simulink model "MainSim"  (R2024a)
(part 10 of 12)

  "IW{1,1}(91,:)'" : Constant  Value=[0.07063741223789991863224457802061806432902812957763671875;-0.08871882270486421140365251858383999206125736236572265625;0.0006579027296117509297779246679738207603804767131805419921875;-0.01173923498918761666731658266371596255339682102203369140625;-0.01047479372654045760848706692058840417303144931793212890625;-0.019136290652363503739241679113547434099018573760986328125;-0.0260832109095130472431467438809704617597162723541259765625;0.0247262166900140654968165421223602606914937496185302734375;-0.0230945968221924653740462218820539419539272785186767578125;-0.00669175803018199656657660767677953117527067661285400390625;-0.02521354944576546797119220855165622197091579437255859375;0.00151431210226198845365808143270669461344368755817413330078125;0.02841805038105411906901309748718631453812122344970703125;0.0267906724159141622354507461523098754696547985076904296875]
      mask Display: e = 0.06;c1 = [120 150 230]/255;c2 = ([120 150 230]+0)/383;c3 = ([120 150 230]+128)/383;patch([0 1 1 0],[0 0 1 1],c1);patch([0 1 1 1-e 1-e 0+e],[0 0 1 1-e 0+e 0+e],c2);patch([0 0 1 1-e 0+e 0+e],[0 1 1 1-e 1-e 0+e],c3);plot([0 1 1 0 0],[0 0 1 1 0]);disp('Weights');
  "IW{1,1}(92,:)'" : Constant  Value=[-0.01208219342854178167401268950698067783378064632415771484375;0.0067192472598249473880738236175602651201188564300537109375;-0.01018004902194633194689732391680081491358578205108642578125;-0.0034201050886383775606613966147051542066037654876708984375;-0.00346664875944259487372534067617380060255527496337890625;0.00407538024919248086097578465114565915428102016448974609375;-0.0001579382642456296005108173918785041678347624838352203369140625;0.004590930287056878278395544157319818623363971710205078125;-0.006531130622358559227602636809706382337026298046112060546875;-0.007838052866014667829919204677935340441763401031494140625;0.01154164356092016695265467518538571312092244625091552734375;-0.00469984162117397137603536094729861360974609851837158203125;0.0053619108677808897944760957443577353842556476593017578125;0.0128726196335035812656766296413479722104966640472412109375]
      mask Display: e = 0.06;c1 = [120 150 230]/255;c2 = ([120 150 230]+0)/383;c3 = ([120 150 230]+128)/383;patch([0 1 1 0],[0 0 1 1],c1);patch([0 1 1 1-e 1-e 0+e],[0 0 1 1-e 0+e 0+e],c2);patch([0 0 1 1-e 0+e 0+e],[0 1 1 1-e 1-e 0+e],c3);plot([0 1 1 0 0],[0 0 1 1 0]);disp('Weights');
  "IW{1,1}(93,:)'" : Constant  Value=[0.00663469289612939223943488542545310338027775287628173828125;-0.0029780897264123393046453269761286719585768878459930419921875;0.005417420119265266113817158810661567258648574352264404296875;0.00455848440464646890990518812714071827940642833709716796875;0.0019560567513700354881633902692783522070385515689849853515625;-0.00565136530838120619557596313597969128750264644622802734375;-0.010249816397415255353475771471494226716458797454833984375;0.00870667414768099001687318150288774631917476654052734375;-0.00642539976546986808803030299941383418627083301544189453125;0.00147365805093719660391615722261349219479598104953765869140625;0.0065425459944154218394629651811555959284305572509765625;0.00208761620669374418912678237347790854983031749725341796875;-0.00134558529696151532757675273188624487374909222126007080078125;0.006577099244312635539788658434190438129007816314697265625]
      mask Display: e = 0.06;c1 = [120 150 230]/255;c2 = ([120 150 230]+0)/383;c3 = ([120 150 230]+128)/383;patch([0 1 1 0],[0 0 1 1],c1);patch([0 1 1 1-e 1-e 0+e],[0 0 1 1-e 0+e 0+e],c2);patch([0 0 1 1-e 0+e 0+e],[0 1 1 1-e 1-e 0+e],c3);plot([0 1 1 0 0],[0 0 1 1 0]);disp('Weights');
  "IW{1,1}(94,:)'" : Constant  Value=[0.0133196975876473978905867312505506561137735843658447265625;-0.002724954991086264190214283331670230836607515811920166015625;-0.01292568993384780352828844485202353098429739475250244140625;-0.00010258642474367216947638004054255134178674779832363128662109375;0.0034192712014378713603068860038547427393496036529541015625;-0.0049133132011409709483107377536725834943354129791259765625;-0.0214623812474793208837642310982118942774832248687744140625;0.023007485850688368100858127718311152420938014984130859375;0.019016587387684143195532016079596360214054584503173828125;0.0058914858069833986320418262039311230182647705078125;0.0019757847315106220019431670920084798126481473445892333984375;0.0001740592937999706885619788376828864784329198300838470458984375;-0.005836771553343969749783060052550354157574474811553955078125;-0.01172118802567679619885954167557429173029959201812744140625]
      mask Display: e = 0.06;c1 = [120 150 230]/255;c2 = ([120 150 230]+0)/383;c3 = ([120 150 230]+128)/383;patch([0 1 1 0],[0 0 1 1],c1);patch([0 1 1 1-e 1-e 0+e],[0 0 1 1-e 0+e 0+e],c2);patch([0 0 1 1-e 0+e 0+e],[0 1 1 1-e 1-e 0+e],c3);plot([0 1 1 0 0],[0 0 1 1 0]);disp('Weights');
  "IW{1,1}(95,:)'" : Constant  Value=[-0.030168984435360361728850620011144201271235942840576171875;-0.00242856335944273242499757969881102326326072216033935546875;0.045366474304561275887603954970472841523587703704833984375;0.0235956203780624991506176257871629786677658557891845703125;0.0088950917664759772407467863786223460920155048370361328125;-0.04038602680676041389862263031318434514105319976806640625;-0.055396583699348807272588857131268014200031757354736328125;0.034673033558393163977573436795864836312830448150634765625;-0.01259596599131877769917053910830873064696788787841796875;0.00887435102632798920863077540843733004294335842132568359375;0.021710772551334543700729540205429657362401485443115234375;-0.01202374062881248449607962669460903271101415157318115234375;-0.00913509215609213144626554736760226660408079624176025390625;0.020010212544438167603377820569221512414515018463134765625]
      mask Display: e = 0.06;c1 = [120 150 230]/255;c2 = ([120 150 230]+0)/383;c3 = ([120 150 230]+128)/383;patch([0 1 1 0],[0 0 1 1],c1);patch([0 1 1 1-e 1-e 0+e],[0 0 1 1-e 0+e 0+e],c2);patch([0 0 1 1-e 0+e 0+e],[0 1 1 1-e 1-e 0+e],c3);plot([0 1 1 0 0],[0 0 1 1 0]);disp('Weights');
  "IW{1,1}(96,:)'" : Constant  Value=[-0.05226400603406648748272544935389305464923381805419921875;0.0273221261562778573728227371475441032089293003082275390625;0.0258205096419121642170591002241053502075374126434326171875;0.0113152954568486972808383228539241827093064785003662109375;-0.0110224380149167890119432655637865536846220493316650390625;-0.0183353680525855343430574606600202969275414943695068359375;-0.018711723571017128964211195807365584187209606170654296875;-0.0173876375265110405532453796695335768163204193115234375;0.00068990722089190830053351266570871302974410355091094970703125;0.02452344814787373039610685054867644794285297393798828125;-0.015917217658364547772098518407801748253405094146728515625;0.0109260537933429692503128904945697286166250705718994140625;0.006101429406713741905587955471901295823045074939727783203125;0.007714180790291681223680431145339753129519522190093994140625]
      mask Display: e = 0.06;c1 = [120 150 230]/255;c2 = ([120 150 230]+0)/383;c3 = ([120 150 230]+128)/383;patch([0 1 1 0],[0 0 1 1],c1);patch([0 1 1 1-e 1-e 0+e],[0 0 1 1-e 0+e 0+e],c2);patch([0 0 1 1-e 0+e 0+e],[0 1 1 1-e 1-e 0+e],c3);plot([0 1 1 0 0],[0 0 1 1 0]);disp('Weights');
  "IW{1,1}(97,:)'" : Constant  Value=[-0.01271120469215512686911306872161731007508933544158935546875;0.0029051811219069716661633773213679887703619897365570068359375;0.0026221018723518560618324091393560593132860958576202392578125;-0.005134367328952889157622774263245446491055190563201904296875;-0.00274391636624273828337639002938885823823511600494384765625;-0.008903427967942099952036727472659549675881862640380859375;-0.01394853375048086228937815889139528735540807247161865234375;0.0161885508909591878390354935390860191546380519866943359375;0.006177978217436277084961826489006853080354630947113037109375;-0.00474236355881050251903641168382819159887731075286865234375;0.0011100417623952272237752847416913937195204198360443115234375;-0.007804969943815354138649809101480059325695037841796875;0.0026443898432858318169047517898206933750770986080169677734375;-0.002549758171897571756847611368357320316135883331298828125]
      mask Display: e = 0.06;c1 = [120 150 230]/255;c2 = ([120 150 230]+0)/383;c3 = ([120 150 230]+128)/383;patch([0 1 1 0],[0 0 1 1],c1);patch([0 1 1 1-e 1-e 0+e],[0 0 1 1-e 0+e 0+e],c2);patch([0 0 1 1-e 0+e 0+e],[0 1 1 1-e 1-e 0+e],c3);plot([0 1 1 0 0],[0 0 1 1 0]);disp('Weights');
  "IW{1,1}(98,:)'" : Constant  Value=[0.01680988917533955684380231332397670485079288482666015625;-0.016287284319194537951513979123774333856999874114990234375;0.006126833448734378580191606289417904918082058429718017578125;0.00891914449581840580727476464062419836409389972686767578125;0.0052329151305931242976754447226994670927524566650390625;-0.0141034774720301403494460146248457022011280059814453125;-0.0241382135885616598558467416069106548093259334564208984375;0.01558620993734481825765403328887259704060852527618408203125;-0.00181381654274688866070042170264287051395513117313385009765625;0.00478300775746385957443163050584189477376639842987060546875;0.00464685931016431581774828174502545152790844440460205078125;0.00166038039346685039297779606926042106351815164089202880859375;0.00118738160556240983541098632514376731705851852893829345703125;0.005989139214336841772479136380979980458505451679229736328125]
      mask Display: e = 0.06;c1 = [120 150 230]/255;c2 = ([120 150 230]+0)/383;c3 = ([120 150 230]+128)/383;patch([0 1 1 0],[0 0 1 1],c1);patch([0 1 1 1-e 1-e 0+e],[0 0 1 1-e 0+e 0+e],c2);patch([0 0 1 1-e 0+e 0+e],[0 1 1 1-e 1-e 0+e],c3);plot([0 1 1 0 0],[0 0 1 1 0]);disp('Weights');
  "IW{1,1}(99,:)'" : Constant  Value=[0.00915866334388989143666659487053038901649415493011474609375;-0.0199881171056931726537353455341872177086770534515380859375;0.0292708625049807914797472818690948770381510257720947265625;0.0273509617718294718857752201301991590298712253570556640625;0.0171598449904944612420809590958015178330242633819580078125;0.00935099324310617076305707229266772628761827945709228515625;0.0188901316024791994518938764713311684317886829376220703125;-0.011542775357101166255890944967177347280085086822509765625;0.014954836457782456904386236828941036947071552276611328125;0.017637024589468898450039802128230803646147251129150390625;-0.0021220429574456164782680911429224579478614032268524169921875;0.0004286890763189841742179797545730934871244244277477264404296875;0.00048205508339510213557110862581112087354995310306549072265625;-0.017889644911831655005318708617778611369431018829345703125]
      mask Display: e = 0.06;c1 = [120 150 230]/255;c2 = ([120 150 230]+0)/383;c3 = ([120 150 230]+128)/383;patch([0 1 1 0],[0 0 1 1],c1);patch([0 1 1 1-e 1-e 0+e],[0 0 1 1-e 0+e 0+e],c2);patch([0 0 1 1-e 0+e 0+e],[0 1 1 1-e 1-e 0+e],c3);plot([0 1 1 0 0],[0 0 1 1 0]);disp('Weights');
  Mux : Mux  Inputs=125
      mask Display: e = 0.06;c1 = [120 150 230]/255;c2 = ([120 150 230]+0)/383;c3 = ([120 150 230]+128)/383;patch([0 1 1 0],[0 0 1 1],c1);patch([0 1 1 1-e 1-e 0+e],[0 0 1 1-e 0+e 0+e],c2);patch([0 0 1 1-e 0+e 0+e],[0 1 1 1-e 1-e 0+e],c3);plot([0 1 1 0 0],[0 0 1 1 0]);disp('Mux');
  dotprod{1..125} (125 alike) : neural/Weight Functions/dotprod
  "iz{1,1}" : Outport
      mask Display: e = 0.06;c1 = [120 230 180]/255;c2 = ([120 230 180]+0)/(256+128);c3 = ([120 230 180]+128)/(256+128);patch([0 1 1 0],[0 0 1 1],c1);patch([0 1 1 1-e 1-e 0+e],[0 0 1 1-e 0+e 0+e],c2);patch([0 0 1 1-e 0+e 0+e],[0 1 1 1-e 1-e 0+e],c3);plot([0 1 1 0 0],[0 0 1 1 0]);
  wires:
  Mux/1 -> "iz{1,1}"/1
  dotprod125/1 -> Mux/125
  "IW{1,1}(125,:)'"/1 -> dotprod125/1
  dotprod124/1 -> Mux/124
  "IW{1,1}(124,:)'"/1 -> dotprod124/1
  dotprod123/1 -> Mux/123
  "IW{1,1}(123,:)'"/1 -> dotprod123/1
  dotprod122/1 -> Mux/122
  "IW{1,1}(122,:)'"/1 -> dotprod122/1
  dotprod121/1 -> Mux/121
  "IW{1,1}(121,:)'"/1 -> dotprod121/1
  dotprod120/1 -> Mux/120
  "IW{1,1}(120,:)'"/1 -> dotprod120/1
  dotprod119/1 -> Mux/119
  "IW{1,1}(119,:)'"/1 -> dotprod119/1
  dotprod118/1 -> Mux/118
  "IW{1,1}(118,:)'"/1 -> dotprod118/1
  dotprod117/1 -> Mux/117
  "IW{1,1}(117,:)'"/1 -> dotprod117/1
  dotprod116/1 -> Mux/116
  "IW{1,1}(116,:)'"/1 -> dotprod116/1
  dotprod115/1 -> Mux/115
  "IW{1,1}(115,:)'"/1 -> dotprod115/1
  dotprod114/1 -> Mux/114
  "IW{1,1}(114,:)'"/1 -> dotprod114/1
  dotprod113/1 -> Mux/113
  "IW{1,1}(113,:)'"/1 -> dotprod113/1
  dotprod112/1 -> Mux/112
  "IW{1,1}(112,:)'"/1 -> dotprod112/1
  dotprod111/1 -> Mux/111
  "IW{1,1}(111,:)'"/1 -> dotprod111/1
  dotprod110/1 -> Mux/110
  "IW{1,1}(110,:)'"/1 -> dotprod110/1
  dotprod109/1 -> Mux/109
  "IW{1,1}(109,:)'"/1 -> dotprod109/1
  dotprod108/1 -> Mux/108
  "IW{1,1}(108,:)'"/1 -> dotprod108/1
  dotprod107/1 -> Mux/107
  "IW{1,1}(107,:)'"/1 -> dotprod107/1
  dotprod106/1 -> Mux/106
  "IW{1,1}(106,:)'"/1 -> dotprod106/1
  dotprod105/1 -> Mux/105
  "IW{1,1}(105,:)'"/1 -> dotprod105/1
  dotprod104/1 -> Mux/104
  "IW{1,1}(104,:)'"/1 -> dotprod104/1
  dotprod103/1 -> Mux/103
  "IW{1,1}(103,:)'"/1 -> dotprod103/1
  dotprod102/1 -> Mux/102
  "IW{1,1}(102,:)'"/1 -> dotprod102/1
  dotprod101/1 -> Mux/101
  "IW{1,1}(101,:)'"/1 -> dotprod101/1
  dotprod100/1 -> Mux/100
  "IW{1,1}(100,:)'"/1 -> dotprod100/1
  dotprod99/1 -> Mux/99
  "IW{1,1}(99,:)'"/1 -> dotprod99/1
  dotprod98/1 -> Mux/98
  "IW{1,1}(98,:)'"/1 -> dotprod98/1
  dotprod97/1 -> Mux/97
  "IW{1,1}(97,:)'"/1 -> dotprod97/1
  dotprod96/1 -> Mux/96
  "IW{1,1}(96,:)'"/1 -> dotprod96/1
  dotprod95/1 -> Mux/95
  "IW{1,1}(95,:)'"/1 -> dotprod95/1
  dotprod94/1 -> Mux/94
  "IW{1,1}(94,:)'"/1 -> dotprod94/1
  dotprod93/1 -> Mux/93
  "IW{1,1}(93,:)'"/1 -> dotprod93/1
  dotprod92/1 -> Mux/92
  "IW{1,1}(92,:)'"/1 -> dotprod92/1
  dotprod91/1 -> Mux/91
  "IW{1,1}(91,:)'"/1 -> dotprod91/1
  dotprod90/1 -> Mux/90
  "IW{1,1}(90,:)'"/1 -> dotprod90/1
  dotprod89/1 -> Mux/89
  "IW{1,1}(89,:)'"/1 -> dotprod89/1
  dotprod88/1 -> Mux/88
  "IW{1,1}(88,:)'"/1 -> dotprod88/1
  dotprod87/1 -> Mux/87
  "IW{1,1}(87,:)'"/1 -> dotprod87/1
  dotprod86/1 -> Mux/86
  "IW{1,1}(86,:)'"/1 -> dotprod86/1
  dotprod85/1 -> Mux/85
  "IW{1,1}(85,:)'"/1 -> dotprod85/1
  dotprod84/1 -> Mux/84
  "IW{1,1}(84,:)'"/1 -> dotprod84/1
  dotprod83/1 -> Mux/83
  "IW{1,1}(83,:)'"/1 -> dotprod83/1
  dotprod82/1 -> Mux/82
  "IW{1,1}(82,:)'"/1 -> dotprod82/1
  dotprod81/1 -> Mux/81
  "IW{1,1}(81,:)'"/1 -> dotprod81/1
  dotprod80/1 -> Mux/80
  "IW{1,1}(80,:)'"/1 -> dotprod80/1
  dotprod79/1 -> Mux/79
  "IW{1,1}(79,:)'"/1 -> dotprod79/1
  dotprod78/1 -> Mux/78
  "IW{1,1}(78,:)'"/1 -> dotprod78/1
  dotprod77/1 -> Mux/77
  "IW{1,1}(77,:)'"/1 -> dotprod77/1
  dotprod76/1 -> Mux/76
  "IW{1,1}(76,:)'"/1 -> dotprod76/1
  dotprod75/1 -> Mux/75
  "IW{1,1}(75,:)'"/1 -> dotprod75/1
  dotprod74/1 -> Mux/74
  "IW{1,1}(74,:)'"/1 -> dotprod74/1
  dotprod73/1 -> Mux/73
  "IW{1,1}(73,:)'"/1 -> dotprod73/1
  dotprod72/1 -> Mux/72
  "IW{1,1}(72,:)'"/1 -> dotprod72/1
  dotprod71/1 -> Mux/71
  "IW{1,1}(71,:)'"/1 -> dotprod71/1
  dotprod70/1 -> Mux/70
  "IW{1,1}(70,:)'"/1 -> dotprod70/1
  dotprod69/1 -> Mux/69
  "IW{1,1}(69,:)'"/1 -> dotprod69/1
  dotprod68/1 -> Mux/68
  "IW{1,1}(68,:)'"/1 -> dotprod68/1
  dotprod67/1 -> Mux/67
  "IW{1,1}(67,:)'"/1 -> dotprod67/1
  dotprod66/1 -> Mux/66
  "IW{1,1}(66,:)'"/1 -> dotprod66/1
  dotprod65/1 -> Mux/65
  "IW{1,1}(65,:)'"/1 -> dotprod65/1
  dotprod64/1 -> Mux/64
  "IW{1,1}(64,:)'"/1 -> dotprod64/1
  dotprod63/1 -> Mux/63
  "IW{1,1}(63,:)'"/1 -> dotprod63/1
  dotprod62/1 -> Mux/62
  "IW{1,1}(62,:)'"/1 -> dotprod62/1
  dotprod61/1 -> Mux/61
  "IW{1,1}(61,:)'"/1 -> dotprod61/1
  dotprod60/1 -> Mux/60
  "IW{1,1}(60,:)'"/1 -> dotprod60/1
  dotprod59/1 -> Mux/59
  "IW{1,1}(59,:)'"/1 -> dotprod59/1
  dotprod58/1 -> Mux/58
  "IW{1,1}(58,:)'"/1 -> dotprod58/1
  dotprod57/1 -> Mux/57
  "IW{1,1}(57,:)'"/1 -> dotprod57/1
  dotprod56/1 -> Mux/56
  "IW{1,1}(56,:)'"/1 -> dotprod56/1
  dotprod55/1 -> Mux/55
  "IW{1,1}(55,:)'"/1 -> dotprod55/1
  dotprod54/1 -> Mux/54
  "IW{1,1}(54,:)'"/1 -> dotprod54/1
  dotprod53/1 -> Mux/53
  "IW{1,1}(53,:)'"/1 -> dotprod53/1
  dotprod52/1 -> Mux/52
  "IW{1,1}(52,:)'"/1 -> dotprod52/1
  dotprod51/1 -> Mux/51
  "IW{1,1}(51,:)'"/1 -> dotprod51/1
  dotprod50/1 -> Mux/50
  "IW{1,1}(50,:)'"/1 -> dotprod50/1
  dotprod49/1 -> Mux/49
  "IW{1,1}(49,:)'"/1 -> dotprod49/1
  dotprod48/1 -> Mux/48
  "IW{1,1}(48,:)'"/1 -> dotprod48/1
  dotprod47/1 -> Mux/47
  "IW{1,1}(47,:)'"/1 -> dotprod47/1
  dotprod46/1 -> Mux/46
  "IW{1,1}(46,:)'"/1 -> dotprod46/1
  dotprod45/1 -> Mux/45
  "IW{1,1}(45,:)'"/1 -> dotprod45/1
  dotprod44/1 -> Mux/44
  "IW{1,1}(44,:)'"/1 -> dotprod44/1
  dotprod43/1 -> Mux/43
  "IW{1,1}(43,:)'"/1 -> dotprod43/1
  dotprod42/1 -> Mux/42
  "IW{1,1}(42,:)'"/1 -> dotprod42/1
  dotprod41/1 -> Mux/41
  "IW{1,1}(41,:)'"/1 -> dotprod41/1
  dotprod40/1 -> Mux/40
  "IW{1,1}(40,:)'"/1 -> dotprod40/1
  dotprod39/1 -> Mux/39
  "IW{1,1}(39,:)'"/1 -> dotprod39/1
  dotprod38/1 -> Mux/38
  "IW{1,1}(38,:)'"/1 -> dotprod38/1
  dotprod37/1 -> Mux/37
  "IW{1,1}(37,:)'"/1 -> dotprod37/1
  dotprod36/1 -> Mux/36
  "IW{1,1}(36,:)'"/1 -> dotprod36/1
  dotprod35/1 -> Mux/35
  "IW{1,1}(35,:)'"/1 -> dotprod35/1
  dotprod34/1 -> Mux/34
  "IW{1,1}(34,:)'"/1 -> dotprod34/1
  dotprod33/1 -> Mux/33
  "IW{1,1}(33,:)'"/1 -> dotprod33/1
  dotprod32/1 -> Mux/32
  "IW{1,1}(32,:)'"/1 -> dotprod32/1
  dotprod31/1 -> Mux/31
  "IW{1,1}(31,:)'"/1 -> dotprod31/1
  dotprod30/1 -> Mux/30
  "IW{1,1}(30,:)'"/1 -> dotprod30/1
  dotprod29/1 -> Mux/29
  "IW{1,1}(29,:)'"/1 -> dotprod29/1
  dotprod28/1 -> Mux/28
  "IW{1,1}(28,:)'"/1 -> dotprod28/1
  dotprod27/1 -> Mux/27
  "IW{1,1}(27,:)'"/1 -> dotprod27/1
  dotprod26/1 -> Mux/26
  "IW{1,1}(26,:)'"/1 -> dotprod26/1
  dotprod25/1 -> Mux/25
  "IW{1,1}(25,:)'"/1 -> dotprod25/1
  dotprod24/1 -> Mux/24
  "IW{1,1}(24,:)'"/1 -> dotprod24/1
  dotprod23/1 -> Mux/23
  "IW{1,1}(23,:)'"/1 -> dotprod23/1
  dotprod22/1 -> Mux/22
  "IW{1,1}(22,:)'"/1 -> dotprod22/1
  dotprod21/1 -> Mux/21
  "IW{1,1}(21,:)'"/1 -> dotprod21/1
  dotprod20/1 -> Mux/20
  "IW{1,1}(20,:)'"/1 -> dotprod20/1
  dotprod19/1 -> Mux/19
  "IW{1,1}(19,:)'"/1 -> dotprod19/1
  dotprod18/1 -> Mux/18
  "IW{1,1}(18,:)'"/1 -> dotprod18/1
  dotprod17/1 -> Mux/17
  "IW{1,1}(17,:)'"/1 -> dotprod17/1
  dotprod16/1 -> Mux/16
  "IW{1,1}(16,:)'"/1 -> dotprod16/1
  dotprod15/1 -> Mux/15
  "IW{1,1}(15,:)'"/1 -> dotprod15/1
  dotprod14/1 -> Mux/14
  "IW{1,1}(14,:)'"/1 -> dotprod14/1
  dotprod13/1 -> Mux/13
  "IW{1,1}(13,:)'"/1 -> dotprod13/1
  dotprod12/1 -> Mux/12
  "IW{1,1}(12,:)'"/1 -> dotprod12/1
  dotprod11/1 -> Mux/11
  "IW{1,1}(11,:)'"/1 -> dotprod11/1
  dotprod10/1 -> Mux/10
  "IW{1,1}(10,:)'"/1 -> dotprod10/1
  dotprod9/1 -> Mux/9
  "IW{1,1}(9,:)'"/1 -> dotprod9/1
  dotprod8/1 -> Mux/8
  "IW{1,1}(8,:)'"/1 -> dotprod8/1
  dotprod7/1 -> Mux/7
  "IW{1,1}(7,:)'"/1 -> dotprod7/1
  dotprod6/1 -> Mux/6
  "IW{1,1}(6,:)'"/1 -> dotprod6/1
  dotprod5/1 -> Mux/5
  "IW{1,1}(5,:)'"/1 -> dotprod5/1
  dotprod4/1 -> Mux/4
  "IW{1,1}(4,:)'"/1 -> dotprod4/1
  dotprod3/1 -> Mux/3
  "IW{1,1}(3,:)'"/1 -> dotprod3/1
  dotprod2/1 -> Mux/2
  "IW{1,1}(2,:)'"/1 -> dotprod2/1
  dotprod1/1 -> Mux/1
  "pd{1,1}"/1 -> dotprod125/2, dotprod124/2, dotprod123/2, dotprod122/2, dotprod121/2, dotprod120/2, dotprod119/2, dotprod118/2, dotprod117/2, dotprod116/2, dotprod115/2, dotprod114/2, dotprod113/2, dotprod112/2, dotprod111/2, dotprod110/2, dotprod109/2, dotprod108/2, dotprod107/2, dotprod106/2, dotprod105/2, dotprod104/2, dotprod103/2, dotprod102/2, dotprod101/2, dotprod100/2, dotprod99/2, dotprod98/2, dotprod97/2, dotprod96/2, dotprod95/2, dotprod94/2, dotprod93/2, dotprod92/2, dotprod91/2, dotprod90/2, dotprod89/2, dotprod88/2, dotprod87/2, dotprod86/2, dotprod85/2, dotprod84/2, dotprod83/2, dotprod82/2, dotprod81/2, dotprod80/2, dotprod79/2, dotprod78/2, dotprod77/2, dotprod76/2, dotprod75/2, dotprod74/2, dotprod73/2, dotprod72/2, dotprod71/2, dotprod70/2, dotprod69/2, dotprod68/2, dotprod67/2, dotprod66/2, dotprod65/2, dotprod64/2, dotprod63/2, dotprod62/2, dotprod61/2, dotprod60/2, dotprod59/2, dotprod58/2, dotprod57/2, dotprod56/2, dotprod55/2, dotprod54/2, dotprod53/2, dotprod52/2, dotprod51/2, dotprod50/2, dotprod49/2, dotprod48/2, dotprod47/2, dotprod46/2, dotprod45/2, dotprod44/2, dotprod43/2, dotprod42/2, dotprod41/2, dotprod40/2, dotprod39/2, dotprod38/2, dotprod37/2, dotprod36/2, dotprod35/2, dotprod34/2, dotprod33/2, dotprod32/2, dotprod31/2, dotprod30/2, dotprod29/2, dotprod28/2, dotprod27/2, dotprod26/2, dotprod25/2, dotprod24/2, dotprod23/2, dotprod22/2, dotprod21/2, dotprod20/2, dotprod19/2, dotprod18/2, dotprod17/2, dotprod16/2, dotprod15/2, dotprod14/2, dotprod13/2, dotprod12/2, dotprod11/2, dotprod10/2, dotprod9/2, dotprod8/2, dotprod7/2, dotprod6/2, dotprod5/2, dotprod4/2, dotprod3/2, dotprod2/2, dotprod1/2
  "IW{1,1}(1,:)'"/1 -> dotprod1/1
